simulink model "EMT_9_bus_1"  (R2023b)
settings: Solver=VariableStepAuto  StartTime=0.0  StopTime=0.2  RelTol=1e-3
libraries: spsSeriesRLCBranchLib x18, spsGroundLib x15, spsThreePhaseParallelRLCBranchLib x12, spsControlledCurrentSourceLib x9, spsThreePhaseVIMeasurementLib x6, spspowerguiLib x1
settings Model: Creator=dongyuli  LastModifiedBy=dongyuli

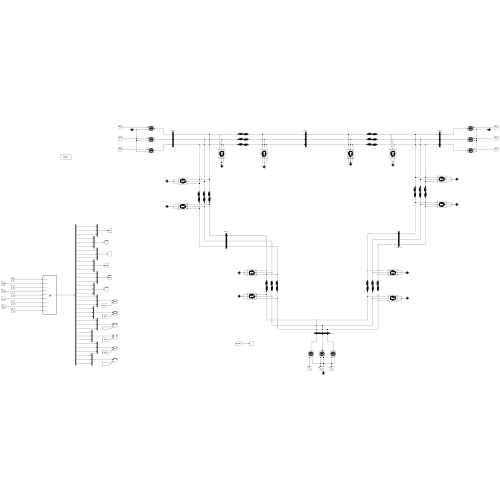
[thumbnail: Simulink's stored preview of the top-level diagram]
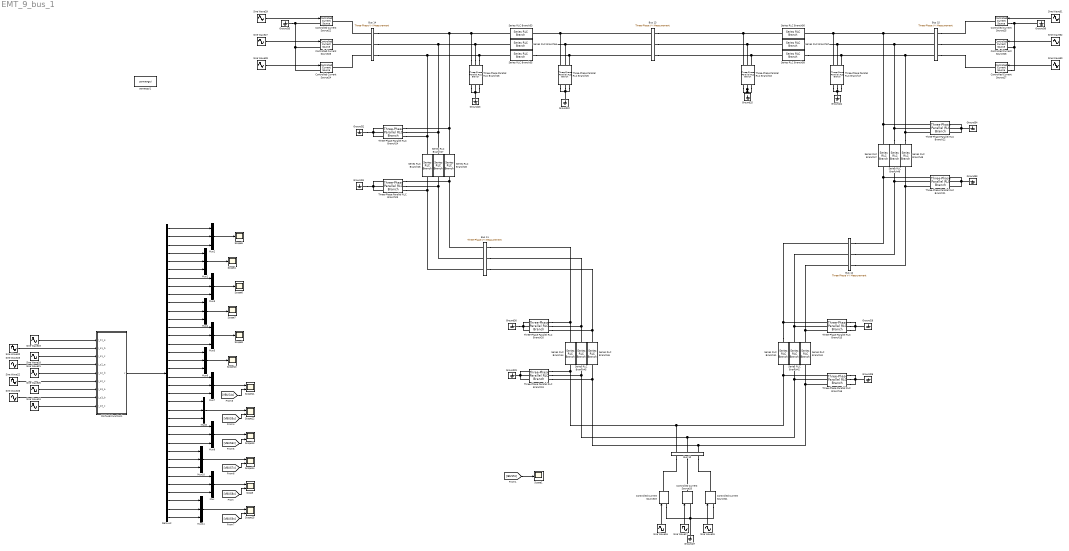
== system EMT_9_bus_1 ==
  Bus 10 : spsThreePhaseVIMeasurementLib/Three-Phase V-I Measurement  VoltageMeasurement=phase-to-ground  SetLabelV=on  LabelV=VBUS4z  Vpu=off  VpuLL=off  CurrentMeasurement=yes  SetLabelI=on  LabelI=IBUS4z  Ipu=off  Pbase=100e6  Vbase=500e3  OutputType=Complex  PhasorSimulation=off  PSBequivalent=0
  Bus 11 : spsThreePhaseVIMeasurementLib/Three-Phase V-I Measurement  VoltageMeasurement=phase-to-ground  SetLabelV=on  LabelV=VBUS5z  Vpu=off  VpuLL=off  CurrentMeasurement=yes  SetLabelI=on  LabelI=IBUS5z  Ipu=off  Pbase=100e6  Vbase=500e3  OutputType=Complex  PhasorSimulation=off  PSBequivalent=0
  Bus 12 : spsThreePhaseVIMeasurementLib/Three-Phase V-I Measurement  VoltageMeasurement=phase-to-ground  SetLabelV=on  LabelV=VBUS6z  Vpu=off  VpuLL=off  CurrentMeasurement=yes  SetLabelI=on  LabelI=IBUS6z  Ipu=off  Pbase=100e6  Vbase=500e3  OutputType=Complex  PhasorSimulation=off  PSBequivalent=0
  Bus 13 : spsThreePhaseVIMeasurementLib/Three-Phase V-I Measurement  VoltageMeasurement=phase-to-ground  SetLabelV=on  LabelV=VBUS8z  Vpu=off  VpuLL=off  CurrentMeasurement=yes  SetLabelI=on  LabelI=IBUS8z  Ipu=off  Pbase=100e6  Vbase=500e3  OutputType=Complex  PhasorSimulation=off  PSBequivalent=0
  Bus 14 : spsThreePhaseVIMeasurementLib/Three-Phase V-I Measurement  VoltageMeasurement=phase-to-ground  SetLabelV=on  LabelV=VBUS7z  Vpu=off  VpuLL=off  CurrentMeasurement=yes  SetLabelI=on  LabelI=IBUS7z  Ipu=off  Pbase=100e6  Vbase=500e3  OutputType=Complex  PhasorSimulation=off  PSBequivalent=0
  Bus 15 : spsThreePhaseVIMeasurementLib/Three-Phase V-I Measurement  VoltageMeasurement=phase-to-ground  SetLabelV=on  LabelV=VBUS9z  Vpu=off  VpuLL=off  CurrentMeasurement=yes  SetLabelI=on  LabelI=IBUS9z  Ipu=off  Pbase=100e6  Vbase=500e3  OutputType=Complex  PhasorSimulation=off  PSBequivalent=0
  Controlled Current Source{19..27} (9 alike) : spsControlledCurrentSourceLib/Controlled Current Source  Initialize=on  Source_Type=AC  Amplitude=0  Phase=0  Frequency=0  Measurements=None
  Demux2 : Demux  Outputs=36
  Ground{22..36} (15 alike) : spsGroundLib/Ground  LConnTagsString=a
  MATLAB Function1 : MATLAB Function  TreatAsAtomicUnit=on
  Mux{,1..11} (12 alike) : Mux  Inputs=3
  Scope{,11..15} (6 alike) : Scope  NumInputPorts=2
  Scope{1,4..7,9..10} (7 alike) : Scope
  Series RLC Branch{26..28,41..49,53..58} (18 alike) : spsSeriesRLCBranchLib/Series RLC Branch  LConnTagsString=__new0  RConnTagsString=__new0  BranchType=RL  Resistance=1  Inductance=1e-3  SetiL0=off  InitialCurrent=0  Capacitance=1e-6  Setx0=off  InitialVoltage=0  Measurements=None
  Sine Wave15 : Sin  Amplitude=10  Frequency=2*pi*50  Phase=4*pi/3  SampleTime=0
  Sine Wave16 : Sin  Amplitude=10  Frequency=2*pi*50  SampleTime=0
  Sine Wave17 : Sin  Amplitude=10  Frequency=2*pi*50  Phase=2*pi/3  SampleTime=0
  Sine Wave18 : Sin  Amplitude=10  Frequency=2*pi*50  Phase=2*pi/3  SampleTime=0
  Sine Wave19 : Sin  Amplitude=10  Frequency=2*pi*50  SampleTime=0
  Sine Wave20 : Sin  Amplitude=10  Frequency=2*pi*50  Phase=-2*pi/3  SampleTime=0
  Sine Wave21 : Sin  Amplitude=5  Frequency=2*pi*50  Phase=-2*pi/3  SampleTime=0
  Sine Wave22 : Sin  Amplitude=5  Frequency=2*pi*50  Phase=2*pi/3  SampleTime=0
  Sine Wave23 : Sin  Amplitude=5  Frequency=2*pi*50  SampleTime=0
  Sine Wave24 : Sin  Amplitude=3  Frequency=2*pi*50  Phase=2*pi/3  SampleTime=0
  Sine Wave25 : Sin  Amplitude=3  Frequency=2*pi*50  SampleTime=0
  Sine Wave26 : Sin  Amplitude=3  Frequency=2*pi*50  Phase=-2*pi/3  SampleTime=0
  Sine Wave27 : Sin  Amplitude=5  Frequency=2*pi*50  Phase=2*pi/3  SampleTime=0
  Sine Wave28 : Sin  Amplitude=5  Frequency=2*pi*50  Phase=4*pi/3  SampleTime=0
  Sine Wave29 : Sin  Amplitude=5  Frequency=2*pi*50  SampleTime=0
  Sine Wave30 : Sin  Amplitude=3  Frequency=2*pi*50  Phase=4*pi/3  SampleTime=0
  Sine Wave31 : Sin  Amplitude=3  Frequency=2*pi*50  SampleTime=0
  Sine Wave32 : Sin  Amplitude=3  Frequency=2*pi*50  Phase=2*pi/3  SampleTime=0
  Three-Phase Parallel RLC Branch{15..26} (12 alike) : spsThreePhaseParallelRLCBranchLib/Three-Phase Parallel RLC Branch  LConnTagsString=A|B|C  RConnTagsString=A|B|C  BranchType=RC  Resistance=1  Inductance=1e-3  Capacitance=1e-6  Measurements=None
  powergui1 : spspowerguiLib/powergui  Priority=1  SimulationMode=Discrete  SampleTime=50e-6  frequency=60  Iterations=50  frequencyindice=0  Pbase=100e6  ErrMax=1e-4  UnitsV=kV  UnitsW=MW  buscounter=0  FunctionMessages=off  echomessages=off  EnableUseOfTLC=off  CurrentSourceSwitches=off  DisableSnubberDevices=off  DisableRonSwitches=off  DisableVfSwitches=off  DisplayEquations=off  AutomaticDiscreteSolvers=off  SolverType=Tustin/Backward Euler (TBE)  Interpol=off  ExternalGateDelay=off  methode=off  Ts=100  x0status=blocks  SPID=on  SwTol=0  HookPort=off  NonlinearTolerance=1e-4  nMaxIteration=100  ContinueOnMaxIteration=off  RestoreLinks=warning  ResistiveCurrentMeasurement=off  Frange=[0:2:500]  Ylog=off  Xlog=on  ShowGrid=off  save=off  variable=ZData  structure=0  ZoomFFT=off  StartTime=0.0  cycles=1  DisplayStyle=1  fundamental=60  FreqAxis=off  MaxFrequency=1000  frequencyindicesteady=1  RmsSteady=1  display=off
  wires:
  Sine Wave19/1 -> MATLAB Function1/1(i_s1_a)
  Sine Wave20/1 -> MATLAB Function1/2(i_s1_b)
  Sine Wave18/1 -> MATLAB Function1/3(i_s1_c)
  Sine Wave23/1 -> MATLAB Function1/4(i_s2_a)
  Sine Wave21/1 -> MATLAB Function1/5(i_s2_b)
  Sine Wave22/1 -> MATLAB Function1/6(i_s2_c)
  Sine Wave25/1 -> MATLAB Function1/7(i_s3_a)
  Sine Wave26/1 -> MATLAB Function1/8(i_s3_b)
  Sine Wave24/1 -> MATLAB Function1/9(i_s3_c)
  MATLAB Function1/1(y) -> Demux2/1
  Demux2/31 -> Mux/1
  Demux2/32 -> Mux/2
  Demux2/33 -> Mux/3
  Sine Wave17/1 -> Controlled Current Source20/1
  Sine Wave15/1 -> Controlled Current Source21/1
  Sine Wave16/1 -> Controlled Current Source19/1
  [IBUS5z] -> Scope1/1
  Sine Wave29/1 -> Controlled Current Source22/1
  Sine Wave27/1 -> Controlled Current Source23/1
  Sine Wave28/1 -> Controlled Current Source24/1
  Sine Wave31/1 -> Controlled Current Source25/1
  Sine Wave30/1 -> Controlled Current Source27/1
  Sine Wave32/1 -> Controlled Current Source26/1
  Mux1/1 -> Scope4/1
  Demux2/6 -> Mux1/3
  Demux2/5 -> Mux1/2
  Demux2/4 -> Mux1/1
  Mux2/1 -> Scope5/1
  Demux2/1 -> Mux2/1
  Demux2/2 -> Mux2/2
  Demux2/3 -> Mux2/3
  Mux3/1 -> Scope6/1
  Demux2/7 -> Mux3/1
  Demux2/8 -> Mux3/2
  Demux2/9 -> Mux3/3
  Mux4/1 -> Scope7/1
  Demux2/10 -> Mux4/1
  Demux2/11 -> Mux4/2
  Demux2/12 -> Mux4/3
  Mux5/1 -> Scope9/1
  Demux2/13 -> Mux5/1
  Demux2/14 -> Mux5/2
  Demux2/15 -> Mux5/3
  Mux6/1 -> Scope10/1
  Demux2/16 -> Mux6/1
  Demux2/17 -> Mux6/2
  Demux2/18 -> Mux6/3
  Mux7/1 -> Scope11/1
  Demux2/19 -> Mux7/1
  Demux2/20 -> Mux7/2
  Demux2/21 -> Mux7/3
  Mux8/1 -> Scope12/1
  Demux2/22 -> Mux8/1
  Demux2/23 -> Mux8/2
  Demux2/24 -> Mux8/3
  Demux2/25 -> Mux9/1
  Demux2/26 -> Mux9/2
  Demux2/27 -> Mux9/3
  Mux/1 -> Scope/1
  Mux10/1 -> Scope14/1
  Demux2/28 -> Mux10/1
  Demux2/29 -> Mux10/2
  Demux2/30 -> Mux10/3
  Mux11/1 -> Scope15/1
  Demux2/34 -> Mux11/1
  Demux2/35 -> Mux11/2
  Demux2/36 -> Mux11/3
  [VBUS8z] -> Scope/2
  [VBUS4z] -> Scope11/2
  [VBUS5z] -> Scope12/2
  Mux9/1 -> Scope13/1
  [VBUS6z] -> Scope13/2
  [VBUS7z] -> Scope14/2
  [VBUS9z] -> Scope15/2
  connections:
  Series RLC Branch43/LConn1 -- Three-Phase Parallel RLC Branch16/LConn3 -- Bus 10/RConn3 -- Three-Phase Parallel RLC Branch19/LConn3 -- Series RLC Branch46/LConn1
  Series RLC Branch41/LConn1 -- Three-Phase Parallel RLC Branch16/LConn1 -- Three-Phase Parallel RLC Branch19/LConn1 -- Series RLC Branch44/LConn1 -- Bus 10/RConn1
  Series RLC Branch42/LConn1 -- Three-Phase Parallel RLC Branch16/LConn2 -- Bus 10/RConn2 -- Three-Phase Parallel RLC Branch19/LConn2 -- Series RLC Branch45/LConn1
  Bus 11/LConn2 -- Three-Phase Parallel RLC Branch20/LConn2 -- Series RLC Branch45/RConn1
  Ground26/LConn1 -- Three-Phase Parallel RLC Branch16/RConn3 -- Three-Phase Parallel RLC Branch16/RConn1 -- Three-Phase Parallel RLC Branch16/RConn2
  Bus 11/LConn3 -- Three-Phase Parallel RLC Branch20/LConn1 -- Series RLC Branch44/RConn1
  Bus 11/LConn1 -- Three-Phase Parallel RLC Branch20/LConn3 -- Series RLC Branch46/RConn1
  Ground29/LConn1 -- Three-Phase Parallel RLC Branch19/RConn1 -- Three-Phase Parallel RLC Branch19/RConn3 -- Three-Phase Parallel RLC Branch19/RConn2
  Ground30/LConn1 -- Three-Phase Parallel RLC Branch20/RConn2 -- Three-Phase Parallel RLC Branch20/RConn1 -- Three-Phase Parallel RLC Branch20/RConn3
  Series RLC Branch41/RConn1 -- Three-Phase Parallel RLC Branch15/LConn1 -- Bus 12/LConn1
  Bus 12/LConn3 -- Three-Phase Parallel RLC Branch15/LConn3 -- Series RLC Branch43/RConn1
  Ground27/LConn1 -- Controlled Current Source21/LConn1 -- Controlled Current Source19/LConn1 -- Controlled Current Source20/LConn1
  Ground28/LConn1 -- Three-Phase Parallel RLC Branch15/RConn2 -- Three-Phase Parallel RLC Branch15/RConn3 -- Three-Phase Parallel RLC Branch15/RConn1
  Bus 12/LConn2 -- Three-Phase Parallel RLC Branch15/LConn2 -- Series RLC Branch42/RConn1
  Bus 10/LConn1 -- Controlled Current Source19/RConn1
  Bus 10/LConn3 -- Controlled Current Source21/RConn1
  Bus 10/LConn2 -- Controlled Current Source20/RConn1
  Three-Phase Parallel RLC Branch26/LConn3 -- Three-Phase Parallel RLC Branch24/LConn3 -- Series RLC Branch26/RConn1 -- Bus 14/LConn1 -- Series RLC Branch55/RConn1
  Three-Phase Parallel RLC Branch21/LConn2 -- Bus 12/RConn2 -- Series RLC Branch48/LConn1
  Three-Phase Parallel RLC Branch21/LConn1 -- Series RLC Branch47/LConn1 -- Bus 12/RConn1
  Bus 13/RConn2 -- Three-Phase Parallel RLC Branch25/LConn2 -- Series RLC Branch54/LConn1
  Series RLC Branch56/LConn1 -- Three-Phase Parallel RLC Branch17/LConn1 -- Bus 15/RConn3 -- Three-Phase Parallel RLC Branch22/LConn1 -- Series RLC Branch47/RConn1
  Series RLC Branch55/LConn1 -- Three-Phase Parallel RLC Branch25/LConn3 -- Bus 13/RConn1
  Bus 11/RConn2 -- Series RLC Branch27/LConn1 -- Three-Phase Parallel RLC Branch23/LConn2
  Three-Phase Parallel RLC Branch26/LConn2 -- Series RLC Branch27/RConn1 -- Three-Phase Parallel RLC Branch24/LConn2 -- Bus 14/LConn2 -- Series RLC Branch54/RConn1
  Bus 11/RConn3 -- Series RLC Branch28/LConn1 -- Three-Phase Parallel RLC Branch23/LConn1
  Series RLC Branch48/RConn1 -- Three-Phase Parallel RLC Branch17/LConn2 -- Series RLC Branch57/LConn1 -- Bus 15/RConn2 -- Three-Phase Parallel RLC Branch22/LConn2
  Three-Phase Parallel RLC Branch21/LConn3 -- Series RLC Branch49/LConn1 -- Bus 12/RConn3
  Three-Phase Parallel RLC Branch26/LConn1 -- Bus 14/LConn3 -- Series RLC Branch28/RConn1 -- Three-Phase Parallel RLC Branch24/LConn1 -- Series RLC Branch53/RConn1
  Ground24/LConn1 -- Three-Phase Parallel RLC Branch17/RConn3 -- Three-Phase Parallel RLC Branch17/RConn1 -- Three-Phase Parallel RLC Branch17/RConn2
  Series RLC Branch57/RConn1 -- Three-Phase Parallel RLC Branch18/LConn2 -- Bus 13/LConn2
  Ground22/LConn1 -- Three-Phase Parallel RLC Branch25/RConn2 -- Three-Phase Parallel RLC Branch25/RConn1 -- Three-Phase Parallel RLC Branch25/RConn3
  Three-Phase Parallel RLC Branch23/LConn3 -- Bus 11/RConn1 -- Series RLC Branch26/LConn1
  Series RLC Branch49/RConn1 -- Three-Phase Parallel RLC Branch17/LConn3 -- Series RLC Branch58/LConn1 -- Bus 15/RConn1 -- Three-Phase Parallel RLC Branch22/LConn3
  Series RLC Branch58/RConn1 -- Three-Phase Parallel RLC Branch18/LConn3 -- Bus 13/LConn1
  Three-Phase Parallel RLC Branch26/RConn2 -- Ground23/LConn1 -- Three-Phase Parallel RLC Branch26/RConn3 -- Three-Phase Parallel RLC Branch26/RConn1
  Ground31/LConn1 -- Three-Phase Parallel RLC Branch23/RConn1 -- Three-Phase Parallel RLC Branch23/RConn3 -- Three-Phase Parallel RLC Branch23/RConn2
  Series RLC Branch56/RConn1 -- Three-Phase Parallel RLC Branch18/LConn1 -- Bus 13/LConn3
  Bus 13/RConn3 -- Three-Phase Parallel RLC Branch25/LConn1 -- Series RLC Branch53/LConn1
  Ground33/LConn1 -- Three-Phase Parallel RLC Branch21/RConn3 -- Three-Phase Parallel RLC Branch21/RConn2 -- Three-Phase Parallel RLC Branch21/RConn1
  Ground34/LConn1 -- Three-Phase Parallel RLC Branch22/RConn3 -- Three-Phase Parallel RLC Branch22/RConn1 -- Three-Phase Parallel RLC Branch22/RConn2
  Ground25/LConn1 -- Three-Phase Parallel RLC Branch18/RConn2 -- Three-Phase Parallel RLC Branch18/RConn3 -- Three-Phase Parallel RLC Branch18/RConn1
  Ground32/LConn1 -- Three-Phase Parallel RLC Branch24/RConn3 -- Three-Phase Parallel RLC Branch24/RConn2 -- Three-Phase Parallel RLC Branch24/RConn1
  Controlled Current Source24/LConn1 -- Controlled Current Source23/LConn1 -- Ground35/LConn1 -- Controlled Current Source22/LConn1
  Bus 14/RConn1 -- Controlled Current Source24/RConn1
  Bus 14/RConn2 -- Controlled Current Source23/RConn1
  Bus 14/RConn3 -- Controlled Current Source22/RConn1
  Ground36/LConn1 -- Controlled Current Source25/LConn1 -- Controlled Current Source27/LConn1 -- Controlled Current Source26/LConn1
  Bus 15/LConn1 -- Controlled Current Source27/RConn1
  Bus 15/LConn3 -- Controlled Current Source25/RConn1
  Bus 15/LConn2 -- Controlled Current Source26/RConn1

== matlab function EMT_9_bus_1/MATLAB Function1 ==
  settings: updateMethod=DISCRETE
  data: i_s1_a input; y output; i_s1_b input; i_s1_c input; i_s2_a input; i_s2_b input; i_s2_c input; i_s3_a input; i_s3_b input; i_s3_c input
function y = fcn(i_s1_a, i_s1_b, i_s1_c, i_s2_a, i_s2_b, i_s2_c, i_s3_a, i_s3_b, i_s3_c)

persistent x_k
persistent x_k1
persistent u_k0
persistent u_k
persistent y_k

if(isempty(x_k))
    x_k = zeros(36,1);
    u_k0 = zeros(9,1);
end

u_k = [i_s1_a, i_s1_b, i_s1_c, i_s2_a, i_s2_b, i_s2_c, i_s3_a, i_s3_b, i_s3_c]';
T = 5e-5;

R45 = 1;
R46 = 1;
R75 = 1;
R78 = 1;
R98 = 1;
R96 = 1;

L45 = 1e-3;
L46 = 1e-3;
L75 = 1e-3;
L78 = 1e-3;
L98 = 1e-3;
L96 = 1e-3;

G4m = 1;
G4n = 1;
G5m = 1;
G5n = 1;
G6m = 1;
G6n = 1;
G7m = 1;
G7n = 1;
G8m = 1;
G8n = 1;
G9m = 1;
G9n = 1;

C4m = 1e-6;
C4n = 1e-6;
C5m = 1e-6;
C5n = 1e-6;
C6m = 1e-6;
C6n = 1e-6;
C7m = 1e-6;
C7n = 1e-6;
C8m = 1e-6;
C8n = 1e-6;
C9m = 1e-6;
C9n = 1e-6;

A = [-R45/L45 0 0 0 0 0 0 0 0 0 0 0 0 0 0 0 0 0 1/L45 0 0 -1/L45 0 0 0 0 0 0 0 0 0 0 0 0 0 0;
     0 -R45/L45 0 0 0 0 0 0 0 0 0 0 0 0 0 0 0 0 0 1/L45 0 0 -1/L45 0 0 0 0 0 0 0 0 0 0 0 0 0;
     0 0 -R45/L45 0 0 0 0 0 0 0 0 0 0 0 0 0 0 0 0 0 1/L45 0 0 -1/L45 0 0 0 0 0 0 0 0 0 0 0 0;
     0 0 0 -R46/L46 0 0 0 0 0 0 0 0 0 0 0 0 0 0 1/L46 0 0 0 0 0 -1/L46 0 0 0 0 0 0 0 0 0 0 0;
     0 0 0 0 -R46/L46 0 0 0 0 0 0 0 0 0 0 0 0 0 0 1/L46 0 0 0 0 0 -1/L46 0 0 0 0 0 0 0 0 0 0;
     0 0 0 0 0 -R46/L46 0 0 0 0 0 0 0 0 0 0 0 0 0 0 1/L46 0 0 0 0 0 -1/L46 0 0 0 0 0 0 0 0 0;
     0 0 0 0 0 0 -R75/L75 0 0 0 0 0 0 0 0 0 0 0 0 0 0 -1/L75 0 0 0 0 0 1/L75 0 0 0 0 0 0 0 0;
     0 0 0 0 0 0 0 -R75/L75 0 0 0 0 0 0 0 0 0 0 0 0 0 0 -1/L75 0 0 0 0 0 1/L75 0 0 0 0 0 0 0;
     0 0 0 0 0 0 0 0 -R75/L75 0 0 0 0 0 0 0 0 0 0 0 0 0 0 -1/L75 0 0 0 0 0 1/L75 0 0 0 0 0 0;
     0 0 0 0 0 0 0 0 0 -R78/L78 0 0 0 0 0 0 0 0 0 0 0 0 0 0 0 0 0 1/L78 0 0 -1/L78 0 0 0 0 0;
     0 0 0 0 0 0 0 0 0 0 -R78/L78 0 0 0 0 0 0 0 0 0 0 0 0 0 0 0 0 0 1/L78 0 0 -1/L78 0 0 0 0;
     0 0 0 0 0 0 0 0 0 0 0 -R78/L78 0 0 0 0 0 0 0 0 0 0 0 0 0 0 0 0 0 1/L78 0 0 -1/L78 0 0 0;
     0 0 0 0 0 0 0 0 0 0 0 0 -R98/L98 0 0 0 0 0 0 0 0 0 0 0 0 0 0 0 0 0 -1/L98 0 0 1/L98 0 0;
     0 0 0 0 0 0 0 0 0 0 0 0 0 -R98/L98 0 0 0 0 0 0 0 0 0 0 0 0 0 0 0 0 0 -1/L98 0 0 1/L98 0;
     0 0 0 0 0 0 0 0 0 0 0 0 0 0 -R98/L98 0 0 0 0 0 0 0 0 0 0 0 0 0 0 0 0 0 -1/L98 0 0 1/L98;
     0 0 0 0 0 0 0 0 0 0 0 0 0 0 0 -R96/L96 0 0 0 0 0 0 0 0 -1/L96 0 0 0 0 0 0 0 0 1/L96 0 0;
     0 0 0 0 0 0 0 0 0 0 0 0 0 0 0 0 -R96/L96 0 0 0 0 0 0 0 0 -1/L96 0 0 0 0 0 0 0 0 1/L96 0;
     0 0 0 0 0 0 0 0 0 0 0 0 0 0 0 0 0 -R96/L96 0 0 0 0 0 0 0 0 -1/L96 0 0 0 0 0 0 0 0 1/L96;
     -1/(C4m+C4n) 0 0 -1/(C4m+C4n) 0 0 0 0 0 0 0 0 0 0 0 0 0 0 -(G4m+G4n)/(C4m+C4n) 0 0 0 0 0 0 0 0 0 0 0 0 0 0 0 0 0;
     0 -1/(C4m+C4n) 0 0 -1/(C4m+C4n) 0 0 0 0 0 0 0 0 0 0 0 0 0 0 -(G4m+G4n)/(C4m+C4n) 0 0 0 0 0 0 0 0 0 0 0 0 0 0 0 0;
     0 0 -1/(C4m+C4n) 0 0 -1/(C4m+C4n) 0 0 0 0 0 0 0 0 0 0 0 0 0 0 -(G4m+G4n)/(C4m+C4n) 0 0 0 0 0 0 0 0 0 0 0 0 0 0 0;
     1/(C5m+C5n) 0 0 0 0 0 1/(C5m+C5n) 0 0 0 0 0 0 0 0 0 0 0 0 0 0 -(G5m+G5n)/(C5m+C5n) 0 0 0 0 0 0 0 0 0 0 0 0 0 0;
     0 1/(C5m+C5n) 0 0 0 0 0 1/(C5m+C5n) 0 0 0 0 0 0 0 0 0 0 0 0 0 0 -(G5m+G5n)/(C5m+C5n) 0 0 0 0 0 0 0 0 0 0 0 0 0;
     0 0 1/(C5m+C5n) 0 0 0 0 0 1/(C5m+C5n) 0 0 0 0 0 0 0 0 0 0 0 0 0 0 -(G5m+G5n)/(C5m+C5n) 0 0 0 0 0 0 0 0 0 0 0 0;
     0 0 0 1/(C6m+C6n) 0 0 0 0 0 0 0 0 0 0 0 1/(C6m+C6n) 0 0 0 0 0 0 0 0 -(G6m+G6n)/(C6m+C6n) 0 0 0 0 0 0 0 0 0 0 0;
     0 0 0 0 1/(C6m+C6n) 0 0 0 0 0 0 0 0 0 0 0 1/(C6m+C6n) 0 0 0 0 0 0 0 0 -(G6m+G6n)/(C6m+C6n) 0 0 0 0 0 0 0 0 0 0;
     0 0 0 0 0 1/(C6m+C6n) 0 0 0 0 0 0 0 0 0 0 0 1/(C6m+C6n) 0 0 0 0 0 0 0 0 -(G6m+G6n)/(C6m+C6n) 0 0 0 0 0 0 0 0 0;
     0 0 0 0 0 0 -1/(C7m+C7n) 0 0 -1/(C7m+C7n) 0 0 0 0 0 0 0 0 0 0 0 0 0 0 0 0 0 -(G7m+G7n)/(C7m+C7n) 0 0 0 0 0 0 0 0;
     0 0 0 0 0 0 0 -1/(C7m+C7n) 0 0 -1/(C7m+C7n) 0 0 0 0 0 0 0 0 0 0 0 0 0 0 0 0 0 -(G7m+G7n)/(C7m+C7n) 0 0 0 0 0 0 0;
     0 0 0 0 0 0 0 0 -1/(C7m+C7n) 0 0 -1/(C7m+C7n) 0 0 0 0 0 0 0 0 0 0 0 0 0 0 0 0 0 -(G7m+G7n)/(C7m+C7n) 0 0 0 0 0 0;
     0 0 0 0 0 0 0 0 0 1/(C8m+C8n) 0 0 1/(C8m+C8n) 0 0 0 0 0 0 0 0 0 0 0 0 0 0 0 0 0 -(G8m+G8n)/(C8m+C8n) 0 0 0 0 0;
     0 0 0 0 0 0 0 0 0 0 1/(C8m+C8n) 0 0 1/(C8m+C8n) 0 0 0 0 0 0 0 0 0 0 0 0 0 0 0 0 0 -(G8m+G8n)/(C8m+C8n) 0 0 0 0;
     0 0 0 0 0 0 0 0 0 0 0 1/(C8m+C8n) 0 0 1/(C8m+C8n) 0 0 0 0 0 0 0 0 0 0 0 0 0 0 0 0 0 -(G8m+G8n)/(C8m+C8n) 0 0 0;
     0 0 0 0 0 0 0 0 0 0 0 0 -1/(C9m+C9n) 0 0 -1/(C9m+C9n) 0 0 0 0 0 0 0 0 0 0 0 0 0 0 0 0 0 -(G9m+G9n)/(C9m+C9n) 0 0;
     0 0 0 0 0 0 0 0 0 0 0 0 0 -1/(C9m+C9n) 0 0 -1/(C9m+C9n) 0 0 0 0 0 0 0 0 0 0 0 0 0 0 0 0 0 -(G9m+G9n)/(C9m+C9n) 0;
     0 0 0 0 0 0 0 0 0 0 0 0 0 0 -1/(C9m+C9n) 0 0 -1/(C9m+C9n) 0 0 0 0 0 0 0 0 0 0 0 0 0 0 0 0 0 -(G9m+G9n)/(C9m+C9n)];

B = [0 0 0 0 0 0 0 0 0;
     0 0 0 0 0 0 0 0 0;
     0 0 0 0 0 0 0 0 0;
     0 0 0 0 0 0 0 0 0;
     0 0 0 0 0 0 0 0 0;
     0 0 0 0 0 0 0 0 0;
     0 0 0 0 0 0 0 0 0;
     0 0 0 0 0 0 0 0 0;
     0 0 0 0 0 0 0 0 0;
     0 0 0 0 0 0 0 0 0;
     0 0 0 0 0 0 0 0 0;
     0 0 0 0 0 0 0 0 0;
     0 0 0 0 0 0 0 0 0;
     0 0 0 0 0 0 0 0 0;
     0 0 0 0 0 0 0 0 0;
     0 0 0 0 0 0 0 0 0;
     0 0 0 0 0 0 0 0 0;
     0 0 0 0 0 0 0 0 0;
     1/(C4m+C4n) 0 0 0 0 0 0 0 0;
     0 1/(C4m+C4n) 0 0 0 0 0 0 0;
     0 0 1/(C4m+C4n) 0 0 0 0 0 0;
     0 0 0 0 0 0 0 0 0;
     0 0 0 0 0 0 0 0 0;
     0 0 0 0 0 0 0 0 0;
     0 0 0 0 0 0 0 0 0;
     0 0 0 0 0 0 0 0 0;
     0 0 0 0 0 0 0 0 0;
     0 0 0 1/(C7m+C7n) 0 0 0 0 0;
     0 0 0 0 1/(C7m+C7n) 0 0 0 0;
     0 0 0 0 0 1/(C7m+C7n) 0 0 0;
     0 0 0 0 0 0 0 0 0;
     0 0 0 0 0 0 0 0 0;
     0 0 0 0 0 0 0 0 0;
     0 0 0 0 0 0 1/(C9m+C9n) 0 0;
     0 0 0 0 0 0 0 1/(C9m+C9n) 0;
     0 0 0 0 0 0 0 0 1/(C9m+C9n)];

C = eye(36);

D = zeros(36,9);

I = eye(36);

A_1 = inv(I-(A*T)/2)*(I+(A*T)/2);
B_1 = inv(I-(A*T)/2)*B*(T/2);
B_2 = inv(I-(A*T)/2)*B*(T/2);
C_1 = C*A_1;
D_1 = C*B_1 + D;
D_2 = C*B_1;

x_k1 = A_1*x_k + B_1*u_k + B_2*u_k0;
y_k = C_1*x_k + D_1*u_k + D_2*u_k0;

x_k = x_k1;
u_k0 = u_k;

y = y_k;

end
